simulink model "mrefrobotarm_modified_previous_y_previous_u_previous_ref_prepro"  (R2018b)
settings: Solver=FixedStepAuto  StartTime=0.0  StopTime=10  RelTol=1e-3  AbsTol=1e-6
undefined symbols (not defined in the file or in its folder): cc, options
libraries: neural x594, simulink x1
(part 10 of 22)

== system mrefrobotarm_modified_previous_y_previous_u_previous_ref_prepro/pre_0.00001/Layer 3/Delays 1 ==
  "p{3}" : Inport  PortDimensions=30
      mask Display: e = 0.06;c1 = [120 230 180]/255;c2 = ([120 230 180]+0)/(256+128);c3 = ([120 230 180]+128)/(256+128);patch([0 1 1 0],[0 0 1 1],c1);patch([0 1 1 1-e 1-e 0+e],[0 0 1 1-e 0+e 0+e],c2);patch([0 0 1 1-e 0+e 0+e],[0 1 1 1-e 1-e 0+e],c3);plot([0 1 1 0 0],[0 0 1 1 0]);
  mux : Mux  Inputs=1
      mask Display: e = 0.06;c1 = [120 150 230]/255;c2 = ([120 150 230]+0)/383;c3 = ([120 150 230]+128)/383;patch([0 1 1 0],[0 0 1 1],c1);patch([0 1 1 1-e 1-e 0+e],[0 0 1 1-e 0+e 0+e],c2);patch([0 0 1 1-e 0+e 0+e],[0 1 1 1-e 1-e 0+e],c3);plot([0 1 1 0 0],[0 0 1 1 0]);disp('Mux')
  "pd{3,2}" : Outport
      mask Display: e = 0.06;c1 = [120 230 180]/255;c2 = ([120 230 180]+0)/(256+128);c3 = ([120 230 180]+128)/(256+128);patch([0 1 1 0],[0 0 1 1],c1);patch([0 1 1 1-e 1-e 0+e],[0 0 1 1-e 0+e 0+e],c2);patch([0 0 1 1-e 0+e 0+e],[0 1 1 1-e 1-e 0+e],c3);plot([0 1 1 0 0],[0 0 1 1 0]);
  wires:
  "p{3}"/1 -> mux/1
  mux/1 -> "pd{3,2}"/1

== system mrefrobotarm_modified_previous_y_previous_u_previous_ref_prepro/pre_0.00001/Layer 3/LW{3,2} ==
  "ad{3,2}" : Inport  PortDimensions=30
      mask Display: e = 0.06;c1 = [120 230 180]/255;c2 = ([120 230 180]+0)/(256+128);c3 = ([120 230 180]+128)/(256+128);patch([0 1 1 0],[0 0 1 1],c1);patch([0 1 1 1-e 1-e 0+e],[0 0 1 1-e 0+e 0+e],c2);patch([0 0 1 1-e 0+e 0+e],[0 1 1 1-e 1-e 0+e],c3);plot([0 1 1 0 0],[0 0 1 1 0]);
  "IW{3,2}(1,:)'" : Constant  Value=[-0.02708099117104183217730195565309259109199047088623046875;-0.036414425339180954421802738352198502980172634124755859375;-0.53579786648775529211974344434565864503383636474609375;0.11467219823347153673243070670650922693312168121337890625;0.460121219342909448801748339974437840282917022705078125;-0.355936329943013329835110880594584159553050994873046875;-0.14997445769222839118128831614740192890167236328125;-0.401359794727670859959545168749173171818256378173828125;0.012080379935268614755017324569053016602993011474609375;-0.0298262408680656510018280869189766235649585723876953125;-0.30471843862437941741205804646597243845462799072265625;0.1635094519253192657526341236007283441722393035888671875;-0.322365045322164756047556011253618635237216949462890625;0.2441242607764374794587780570509494282305240631103515625;0.05360123386870309369900411411435925401747226715087890625;0.048342927129308037315080781581855262629687786102294921875;0.4674318676620703438828741127508692443370819091796875;-0.11851143462209069723289900366580695845186710357666015625;0.14037975115201273279552651729318313300609588623046875;-0.415865215452181635757966660094098187983036041259765625;-0.42716646209657971322570801930851303040981292724609375;-0.381889610047790262203903921545133925974369049072265625;0.145833587060073599506182517870911397039890289306640625;-0.2441832694725563357440734080228139646351337432861328125;-0.22157671356331276601991930874646641314029693603515625;0.319918117660031697813138862329651601612567901611328125;-0.528575828850534445990660969982855021953582763671875;-0.417695234753292510276878601871430873870849609375;-0.0213015001949658951130306405730152619071304798126220703125;-0.427062730500115728116128366309567354619503021240234375]
      mask Display: e = 0.06;c1 = [120 150 230]/255;c2 = ([120 150 230]+0)/383;c3 = ([120 150 230]+128)/383;patch([0 1 1 0],[0 0 1 1],c1);patch([0 1 1 1-e 1-e 0+e],[0 0 1 1-e 0+e 0+e],c2);patch([0 0 1 1-e 0+e 0+e],[0 1 1 1-e 1-e 0+e],c3);plot([0 1 1 0 0],[0 0 1 1 0]);disp('weights');
  Mux : Mux  Inputs=1
      mask Display: e = 0.06;c1 = [120 150 230]/255;c2 = ([120 150 230]+0)/383;c3 = ([120 150 230]+128)/383;patch([0 1 1 0],[0 0 1 1],c1);patch([0 1 1 1-e 1-e 0+e],[0 0 1 1-e 0+e 0+e],c2);patch([0 0 1 1-e 0+e 0+e],[0 1 1 1-e 1-e 0+e],c3);plot([0 1 1 0 0],[0 0 1 1 0]);disp('Mux');
  dotprod1 : neural/Weight Functions/dotprod
  "lz{3,2}" : Outport
      mask Display: e = 0.06;c1 = [120 230 180]/255;c2 = ([120 230 180]+0)/(256+128);c3 = ([120 230 180]+128)/(256+128);patch([0 1 1 0],[0 0 1 1],c1);patch([0 1 1 1-e 1-e 0+e],[0 0 1 1-e 0+e 0+e],c2);patch([0 0 1 1-e 0+e 0+e],[0 1 1 1-e 1-e 0+e],c3);plot([0 1 1 0 0],[0 0 1 1 0]);
  wires:
  "IW{3,2}(1,:)'"/1 -> dotprod1/1
  "ad{3,2}"/1 -> dotprod1/2
  dotprod1/1 -> Mux/1
  Mux/1 -> "lz{3,2}"/1

== system mrefrobotarm_modified_previous_y_previous_u_previous_ref_prepro/pre_0.00002/Layer 1/Delays 1 ==
  "p{1}" : Inport  PortDimensions=10
      mask Display: e = 0.06;c1 = [120 230 180]/255;c2 = ([120 230 180]+0)/(256+128);c3 = ([120 230 180]+128)/(256+128);patch([0 1 1 0],[0 0 1 1],c1);patch([0 1 1 1-e 1-e 0+e],[0 0 1 1-e 0+e 0+e],c2);patch([0 0 1 1-e 0+e 0+e],[0 1 1 1-e 1-e 0+e],c3);plot([0 1 1 0 0],[0 0 1 1 0]);
  mux : Mux  Inputs=1
      mask Display: e = 0.06;c1 = [120 150 230]/255;c2 = ([120 150 230]+0)/383;c3 = ([120 150 230]+128)/383;patch([0 1 1 0],[0 0 1 1],c1);patch([0 1 1 1-e 1-e 0+e],[0 0 1 1-e 0+e 0+e],c2);patch([0 0 1 1-e 0+e 0+e],[0 1 1 1-e 1-e 0+e],c3);plot([0 1 1 0 0],[0 0 1 1 0]);disp('Mux')
  "pd{1,1}" : Outport
      mask Display: e = 0.06;c1 = [120 230 180]/255;c2 = ([120 230 180]+0)/(256+128);c3 = ([120 230 180]+128)/(256+128);patch([0 1 1 0],[0 0 1 1],c1);patch([0 1 1 1-e 1-e 0+e],[0 0 1 1-e 0+e 0+e],c2);patch([0 0 1 1-e 0+e 0+e],[0 1 1 1-e 1-e 0+e],c3);plot([0 1 1 0 0],[0 0 1 1 0]);
  wires:
  "p{1}"/1 -> mux/1
  mux/1 -> "pd{1,1}"/1

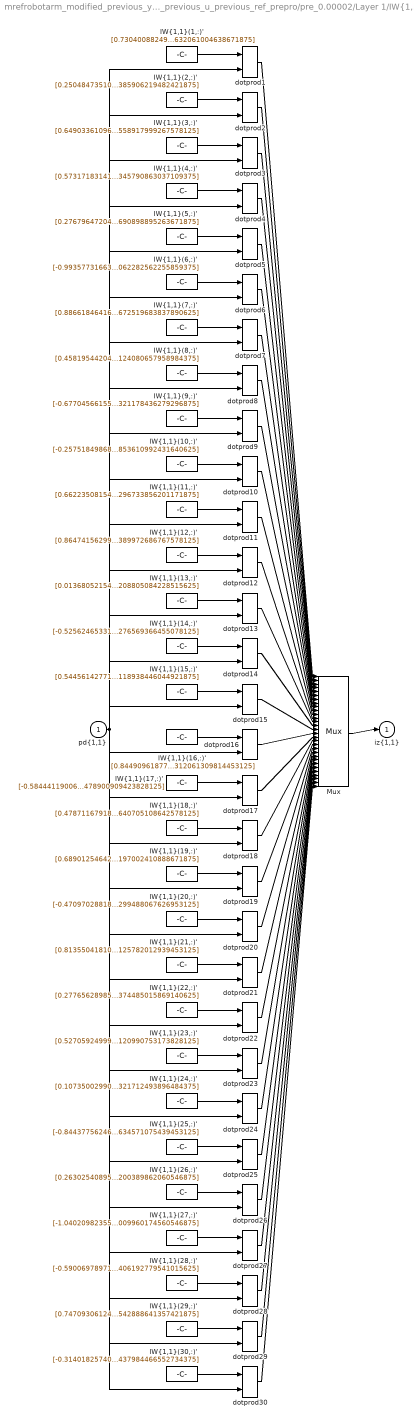
== system mrefrobotarm_modified_previous_y_previous_u_previous_ref_prepro/pre_0.00002/Layer 1/IW{1,1} ==
  "pd{1,1}" : Inport  PortDimensions=10
      mask Display: e = 0.06;c1 = [120 230 180]/255;c2 = ([120 230 180]+0)/(256+128);c3 = ([120 230 180]+128)/(256+128);patch([0 1 1 0],[0 0 1 1],c1);patch([0 1 1 1-e 1-e 0+e],[0 0 1 1-e 0+e 0+e],c2);patch([0 0 1 1-e 0+e 0+e],[0 1 1 1-e 1-e 0+e],c3);plot([0 1 1 0 0],[0 0 1 1 0]);
  "IW{1,1}(1,:)'" : Constant  Value=[0.7304008824925178888776144958683289587497711181640625;0.55735729031188718796130388000165112316608428955078125;-0.274224224023352614043602670790278352797031402587890625;-0.622697954402676057128473985358141362667083740234375;1.191884331831804200163560381042771041393280029296875;-0.67258994734308907847974978722049854695796966552734375;-0.6783417737224137766816056682728230953216552734375;-0.246919049844299520746204734678030945360660552978515625;-0.61337591608532349152227425292949192225933074951171875;-0.60088279688646906162574623522232286632061004638671875]
      mask Display: e = 0.06;c1 = [120 150 230]/255;c2 = ([120 150 230]+0)/383;c3 = ([120 150 230]+128)/383;patch([0 1 1 0],[0 0 1 1],c1);patch([0 1 1 1-e 1-e 0+e],[0 0 1 1-e 0+e 0+e],c2);patch([0 0 1 1-e 0+e 0+e],[0 1 1 1-e 1-e 0+e],c3);plot([0 1 1 0 0],[0 0 1 1 0]);disp('Weights');
  "IW{1,1}(10,:)'" : Constant  Value=[-0.257518498683862950837664129721815697848796844482421875;-0.11405027507294308863894372052527614869177341461181640625;-0.4519201843110665084424226733972318470478057861328125;-0.384415211671115641944851404332439415156841278076171875;-0.356503517164612981904525668142014183104038238525390625;0.9258507361392871448657615474076010286808013916015625;-0.86655442230715185036871162083116360008716583251953125;0.61431897984137495694056951833772473037242889404296875;0.458598179542420825161030961680808104574680328369140625;0.4425235678833419061817266992875374853610992431640625]
      mask Display: e = 0.06;c1 = [120 150 230]/255;c2 = ([120 150 230]+0)/383;c3 = ([120 150 230]+128)/383;patch([0 1 1 0],[0 0 1 1],c1);patch([0 1 1 1-e 1-e 0+e],[0 0 1 1-e 0+e 0+e],c2);patch([0 0 1 1-e 0+e 0+e],[0 1 1 1-e 1-e 0+e],c3);plot([0 1 1 0 0],[0 0 1 1 0]);disp('Weights');
  "IW{1,1}(11,:)'" : Constant  Value=[0.66223508154602706010649626477970741689205169677734375;-0.448412675292931994786016502985148690640926361083984375;0.83225908909172952032662351484759710729122161865234375;0.426264912161532449896839125358383171260356903076171875;0.6714719379842970514715716490172781050205230712890625;-0.5465042912343280878673112965770997107028961181640625;-0.05809258706369181679551871866351575590670108795166015625;-0.8415470336572987708478876811568625271320343017578125;-0.65915992475788309779005658128880895674228668212890625;-0.11957509036706519267578840981514076702296733856201171875]
      mask Display: e = 0.06;c1 = [120 150 230]/255;c2 = ([120 150 230]+0)/383;c3 = ([120 150 230]+128)/383;patch([0 1 1 0],[0 0 1 1],c1);patch([0 1 1 1-e 1-e 0+e],[0 0 1 1-e 0+e 0+e],c2);patch([0 0 1 1-e 0+e 0+e],[0 1 1 1-e 1-e 0+e],c3);plot([0 1 1 0 0],[0 0 1 1 0]);disp('Weights');
  "IW{1,1}(12,:)'" : Constant  Value=[0.8647415629915180534936780532007105648517608642578125;0.367581229875802384388094878886477090418338775634765625;-0.59028723730554644166801381288678385317325592041015625;-0.62213624516392174168544215717702172696590423583984375;-0.623824016499044287087372140376828610897064208984375;0.504078517565071049233438316150568425655364990234375;-0.70493815736031162355601509261759929358959197998046875;-0.66348746327245378129333630567998625338077545166015625;0.28462536860450959874668797056074254214763641357421875;-0.03806284371844066705126152783122961409389972686767578125]
      mask Display: e = 0.06;c1 = [120 150 230]/255;c2 = ([120 150 230]+0)/383;c3 = ([120 150 230]+128)/383;patch([0 1 1 0],[0 0 1 1],c1);patch([0 1 1 1-e 1-e 0+e],[0 0 1 1-e 0+e 0+e],c2);patch([0 0 1 1-e 0+e 0+e],[0 1 1 1-e 1-e 0+e],c3);plot([0 1 1 0 0],[0 0 1 1 0]);disp('Weights');
  "IW{1,1}(13,:)'" : Constant  Value=[0.0136805215469812425921336540568518103100359439849853515625;-0.34441505779833148093160843927762471139430999755859375;1.0216982880331426652986692715785466134548187255859375;0.2435027042613311099028550188450026325881481170654296875;0.34766871164740809074800154121476225554943084716796875;0.624162933978758882602733137900941073894500732421875;0.6576120651417929341420176569954492151737213134765625;0.7039052895761155337339687321218661963939666748046875;-0.6525688408982965871274473101948387920856475830078125;-0.77884807903645114635082791210152208805084228515625]
      mask Display: e = 0.06;c1 = [120 150 230]/255;c2 = ([120 150 230]+0)/383;c3 = ([120 150 230]+128)/383;patch([0 1 1 0],[0 0 1 1],c1);patch([0 1 1 1-e 1-e 0+e],[0 0 1 1-e 0+e 0+e],c2);patch([0 0 1 1-e 0+e 0+e],[0 1 1 1-e 1-e 0+e],c3);plot([0 1 1 0 0],[0 0 1 1 0]);disp('Weights');
  "IW{1,1}(14,:)'" : Constant  Value=[-0.5256246533137678422775707076652906835079193115234375;0.7114248951113688601566309444024227559566497802734375;0.75946178060658031672147671997663564980030059814453125;0.488034362594031267956751207748311571776866912841796875;0.307774644334204150464273652687552385032176971435546875;1.17777346771161273153438742156140506267547607421875;-1.060571928032192801083510858006775379180908203125;-0.8649891627355097423190954941674135625362396240234375;-0.07488935386397999049989948616712354123592376708984375;0.47549822229369731463322068520938046276569366455078125]
      mask Display: e = 0.06;c1 = [120 150 230]/255;c2 = ([120 150 230]+0)/383;c3 = ([120 150 230]+128)/383;patch([0 1 1 0],[0 0 1 1],c1);patch([0 1 1 1-e 1-e 0+e],[0 0 1 1-e 0+e 0+e],c2);patch([0 0 1 1-e 0+e 0+e],[0 1 1 1-e 1-e 0+e],c3);plot([0 1 1 0 0],[0 0 1 1 0]);disp('Weights');
  "IW{1,1}(15,:)'" : Constant  Value=[0.54456142771591242723872028363985009491443634033203125;0.1924337675434008299024668531274073757231235504150390625;0.1103372802512005979025389024172909557819366455078125;0.366407819941435786148531406070105731487274169921875;2.13415426335682933967063945601694285869598388671875;-1.571152442476574151442036963999271392822265625;0.87951877890999152764806012783083133399486541748046875;0.059551333168809457430104004060922306962311267852783203125;0.06808296663973219253751523183382232673466205596923828125;0.31540879799017040863162719688261859118938446044921875]
      mask Display: e = 0.06;c1 = [120 150 230]/255;c2 = ([120 150 230]+0)/383;c3 = ([120 150 230]+128)/383;patch([0 1 1 0],[0 0 1 1],c1);patch([0 1 1 1-e 1-e 0+e],[0 0 1 1-e 0+e 0+e],c2);patch([0 0 1 1-e 0+e 0+e],[0 1 1 1-e 1-e 0+e],c3);plot([0 1 1 0 0],[0 0 1 1 0]);disp('Weights');
  "IW{1,1}(16,:)'" : Constant  Value=[0.8449096187701414795157006665249355137348175048828125;-0.74746261915909906203836499116732738912105560302734375;0.329952307077657158718153596055344678461551666259765625;0.8260485994065922543683200274244882166385650634765625;0.54075535587794931746685733742197044193744659423828125;1.7436566173639054255772862234152853488922119140625;-0.1463094264313840875413319508879794739186763763427734375;-0.660820573047626425022826879285275936126708984375;-0.06815574103313228049305649847156018950045108795166015625;0.42592880572693747609491765615530312061309814453125]
      mask Display: e = 0.06;c1 = [120 150 230]/255;c2 = ([120 150 230]+0)/383;c3 = ([120 150 230]+128)/383;patch([0 1 1 0],[0 0 1 1],c1);patch([0 1 1 1-e 1-e 0+e],[0 0 1 1-e 0+e 0+e],c2);patch([0 0 1 1-e 0+e 0+e],[0 1 1 1-e 1-e 0+e],c3);plot([0 1 1 0 0],[0 0 1 1 0]);disp('Weights');
  "IW{1,1}(17,:)'" : Constant  Value=[-0.58444119006608763466914524542517028748989105224609375;-0.80689482797726075347100049839355051517486572265625;-0.21128881566034196648473653112887404859066009521484375;0.1993104800768525641796458103272016160190105438232421875;0.7910371685352901582888307530083693563938140869140625;-1.6374659717699844296845412827678956091403961181640625;0.2347058211055967069658123591580078937113285064697265625;-0.316128742752765978796247736681834794580936431884765625;0.0220931580819457261399829661741023301146924495697021484375;0.50710898397081038968536859101732261478900909423828125]
      mask Display: e = 0.06;c1 = [120 150 230]/255;c2 = ([120 150 230]+0)/383;c3 = ([120 150 230]+128)/383;patch([0 1 1 0],[0 0 1 1],c1);patch([0 1 1 1-e 1-e 0+e],[0 0 1 1-e 0+e 0+e],c2);patch([0 0 1 1-e 0+e 0+e],[0 1 1 1-e 1-e 0+e],c3);plot([0 1 1 0 0],[0 0 1 1 0]);disp('Weights');
  "IW{1,1}(18,:)'" : Constant  Value=[0.478711679183998206621453164189006201922893524169921875;-0.6843316515233277552709978408529423177242279052734375;0.58763716442424451802395424238056875765323638916015625;0.67534649893978448975673245513462461531162261962890625;-1.089531552775316658454585194704122841358184814453125;1.1625260678634479205584284500218927860260009765625;0.58469035382791589849915681043057702481746673583984375;0.10013888820124013101509063972116564400494098663330078125;-0.78463798649333116319581904463120736181735992431640625;-0.65112497301214411482561672528390772640705108642578125]
      mask Display: e = 0.06;c1 = [120 150 230]/255;c2 = ([120 150 230]+0)/383;c3 = ([120 150 230]+128)/383;patch([0 1 1 0],[0 0 1 1],c1);patch([0 1 1 1-e 1-e 0+e],[0 0 1 1-e 0+e 0+e],c2);patch([0 0 1 1-e 0+e 0+e],[0 1 1 1-e 1-e 0+e],c3);plot([0 1 1 0 0],[0 0 1 1 0]);disp('Weights');
  "IW{1,1}(19,:)'" : Constant  Value=[0.689012546428803052123157613095827400684356689453125;-0.047229633595688429170689204283917206339538097381591796875;-0.7243675903009723082703885665978305041790008544921875;0.1993048568244606411070662943529896438121795654296875;-0.31650746445339195123125364261795766651630401611328125;0.822948088279580769466292622382752597332000732421875;0.98922181344819126724843272313592024147510528564453125;0.440776909161637975298475566887645982205867767333984375;-0.88029002172244386059674070565961301326751708984375;-0.314501274632482619164619563889573328197002410888671875]
      mask Display: e = 0.06;c1 = [120 150 230]/255;c2 = ([120 150 230]+0)/383;c3 = ([120 150 230]+128)/383;patch([0 1 1 0],[0 0 1 1],c1);patch([0 1 1 1-e 1-e 0+e],[0 0 1 1-e 0+e 0+e],c2);patch([0 0 1 1-e 0+e 0+e],[0 1 1 1-e 1-e 0+e],c3);plot([0 1 1 0 0],[0 0 1 1 0]);disp('Weights');
  "IW{1,1}(2,:)'" : Constant  Value=[0.25048473510027247090903301796060986816883087158203125;-1.0819345400682920388391039523412473499774932861328125;0.84795876175950513076173820081748999655246734619140625;-0.56312297055498350406566032688715495169162750244140625;-0.45823196200243498932280772351077757775783538818359375;0.1609611189829285304853101479238830506801605224609375;0.9208277384343850346937188078300096094608306884765625;0.046244571997199612756190845175296999514102935791015625;0.7151359877845873125323805652442388236522674560546875;-0.363929879968436231774120415138895623385906219482421875]
      mask Display: e = 0.06;c1 = [120 150 230]/255;c2 = ([120 150 230]+0)/383;c3 = ([120 150 230]+128)/383;patch([0 1 1 0],[0 0 1 1],c1);patch([0 1 1 1-e 1-e 0+e],[0 0 1 1-e 0+e 0+e],c2);patch([0 0 1 1-e 0+e 0+e],[0 1 1 1-e 1-e 0+e],c3);plot([0 1 1 0 0],[0 0 1 1 0]);disp('Weights');
  "IW{1,1}(20,:)'" : Constant  Value=[-0.47097028818942165973027158543118275701999664306640625;0.74309036858321697582852038976852782070636749267578125;-0.553976745551350457930084303370676934719085693359375;0.033889115275527535720012650699572986923158168792724609375;0.364869656293961508453094211290590465068817138671875;0.410145163811602930792332699638791382312774658203125;-0.2345107364438836217157557939572143368422985076904296875;-0.54322703205234412759949691462679766118526458740234375;0.1590784487766848942502662112019606865942478179931640625;-0.383833262476066583435141410518554039299488067626953125]
      mask Display: e = 0.06;c1 = [120 150 230]/255;c2 = ([120 150 230]+0)/383;c3 = ([120 150 230]+128)/383;patch([0 1 1 0],[0 0 1 1],c1);patch([0 1 1 1-e 1-e 0+e],[0 0 1 1-e 0+e 0+e],c2);patch([0 0 1 1-e 0+e 0+e],[0 1 1 1-e 1-e 0+e],c3);plot([0 1 1 0 0],[0 0 1 1 0]);disp('Weights');
  "IW{1,1}(21,:)'" : Constant  Value=[0.81355041810238504229602085615624673664569854736328125;-1.1474633075534554915719809287111274898052215576171875;0.796433568812742631592982434085570275783538818359375;-0.53342796022723260040976356322062201797962188720703125;0.2163303690425346648140703109675087034702301025390625;-0.053740994151761929675803486361473915167152881622314453125;-0.7139248086813463345379204838536679744720458984375;-0.36399888500070876062864044797606766223907470703125;0.6045317614051251009499310384853743016719818115234375;0.08818159555106726277262652047284063883125782012939453125]
      mask Display: e = 0.06;c1 = [120 150 230]/255;c2 = ([120 150 230]+0)/383;c3 = ([120 150 230]+128)/383;patch([0 1 1 0],[0 0 1 1],c1);patch([0 1 1 1-e 1-e 0+e],[0 0 1 1-e 0+e 0+e],c2);patch([0 0 1 1-e 0+e 0+e],[0 1 1 1-e 1-e 0+e],c3);plot([0 1 1 0 0],[0 0 1 1 0]);disp('Weights');
  "IW{1,1}(22,:)'" : Constant  Value=[0.2776562898561787395834699054830707609653472900390625;-1.2287554150803090546872908817022107541561126708984375;0.0209047426415454491721579444174494710750877857208251953125;0.000445490992757326966476616458834314471459947526454925537109375;1.0480957638323007419245413984754122793674468994140625;-0.07403841976945002567589426689664833247661590576171875;-0.37438154479052376810699342968291603028774261474609375;-0.52846064882596965883720940837520174682140350341796875;0.415750687036309296562563986299210228025913238525390625;0.85104284168978028279894942897954024374485015869140625]
      mask Display: e = 0.06;c1 = [120 150 230]/255;c2 = ([120 150 230]+0)/383;c3 = ([120 150 230]+128)/383;patch([0 1 1 0],[0 0 1 1],c1);patch([0 1 1 1-e 1-e 0+e],[0 0 1 1-e 0+e 0+e],c2);patch([0 0 1 1-e 0+e 0+e],[0 1 1 1-e 1-e 0+e],c3);plot([0 1 1 0 0],[0 0 1 1 0]);disp('Weights');
  "IW{1,1}(23,:)'" : Constant  Value=[0.52705924999088493709820113508612848818302154541015625;0.0660054220044097583741660173473064787685871124267578125;-1.36875726794443952627489125006832182407379150390625;0.311968753379823604543474857564433477818965911865234375;-0.46009367922534283312785419184365309774875640869140625;-0.481466025254796925469946700104628689587116241455078125;-0.3329466073938880388283223510370589792728424072265625;0.1974229762788315689636675642759655602276325225830078125;-1.1254391851952505465561671371688134968280792236328125;-0.9640440286026532579199965766747482120990753173828125]
      mask Display: e = 0.06;c1 = [120 150 230]/255;c2 = ([120 150 230]+0)/383;c3 = ([120 150 230]+128)/383;patch([0 1 1 0],[0 0 1 1],c1);patch([0 1 1 1-e 1-e 0+e],[0 0 1 1-e 0+e 0+e],c2);patch([0 0 1 1-e 0+e 0+e],[0 1 1 1-e 1-e 0+e],c3);plot([0 1 1 0 0],[0 0 1 1 0]);disp('Weights');
  "IW{1,1}(24,:)'" : Constant  Value=[0.10735002990849211446100497369116055779159069061279296875;0.1288206058417812605032537476290599443018436431884765625;0.788111618675113145826571781071834266185760498046875;0.64028048347422850117283132931333966553211212158203125;-0.433917129931848444268638331777765415608882904052734375;0.5940663745965399922255301135010085999965667724609375;1.12816027899131920975150933372788131237030029296875;0.112385069453518282589499222012818790972232818603515625;0.024179242542832761475590785948952543549239635467529296875;0.463315765300100268486716004190384410321712493896484375]
      mask Display: e = 0.06;c1 = [120 150 230]/255;c2 = ([120 150 230]+0)/383;c3 = ([120 150 230]+128)/383;patch([0 1 1 0],[0 0 1 1],c1);patch([0 1 1 1-e 1-e 0+e],[0 0 1 1-e 0+e 0+e],c2);patch([0 0 1 1-e 0+e 0+e],[0 1 1 1-e 1-e 0+e],c3);plot([0 1 1 0 0],[0 0 1 1 0]);disp('Weights');
  "IW{1,1}(25,:)'" : Constant  Value=[-0.84437756246050066355479657431715168058872222900390625;-0.0846648540292919415950478878585272468626499176025390625;0.18704027349657670331595227253274060785770416259765625;-0.2898728359229156836818219744600355625152587890625;-1.09397119609031445719438124797306954860687255859375;-0.44686289863698658297863630650681443512439727783203125;-0.89946061161813783968455027206800878047943115234375;0.636115631845411311218185801408253610134124755859375;0.061844671970694618801100972405038191936910152435302734375;0.17568172897040501556631397761520929634571075439453125]
      mask Display: e = 0.06;c1 = [120 150 230]/255;c2 = ([120 150 230]+0)/383;c3 = ([120 150 230]+128)/383;patch([0 1 1 0],[0 0 1 1],c1);patch([0 1 1 1-e 1-e 0+e],[0 0 1 1-e 0+e 0+e],c2);patch([0 0 1 1-e 0+e 0+e],[0 1 1 1-e 1-e 0+e],c3);plot([0 1 1 0 0],[0 0 1 1 0]);disp('Weights');
  "IW{1,1}(26,:)'" : Constant  Value=[0.26302540895656945085789857330382801592350006103515625;-0.3606987416329634488221245192107744514942169189453125;-0.52244731928137699838998742052353918552398681640625;-0.0285817138234593405565764356879299157299101352691650390625;-0.436131655659286410209318773922859691083431243896484375;1.1469446426500125024716680854908190667629241943359375;0.80450112209670876506351078205625526607036590576171875;0.30490732299961365026064186167786829173564910888671875;-0.50300669421127974789698100721579976379871368408203125;-0.71714061620181535072759970717015676200389862060546875]
      mask Display: e = 0.06;c1 = [120 150 230]/255;c2 = ([120 150 230]+0)/383;c3 = ([120 150 230]+128)/383;patch([0 1 1 0],[0 0 1 1],c1);patch([0 1 1 1-e 1-e 0+e],[0 0 1 1-e 0+e 0+e],c2);patch([0 0 1 1-e 0+e 0+e],[0 1 1 1-e 1-e 0+e],c3);plot([0 1 1 0 0],[0 0 1 1 0]);disp('Weights');
  "IW{1,1}(27,:)'" : Constant  Value=[-1.040209823554227863695587075199000537395477294921875;0.2194302039461969167088994936420931480824947357177734375;-0.528908307700870050638286556932143867015838623046875;-0.478955296274611808104992860535276122391223907470703125;1.0535535961804505244998608759487979114055633544921875;0.1624369124767082173121934829396195709705352783203125;-0.4332507443024322668634340516291558742523193359375;-0.104280016056704283311518111077020876109600067138671875;-0.73485800356468755634153922073892317712306976318359375;-0.50523587261920777091717127404990606009960174560546875]
      mask Display: e = 0.06;c1 = [120 150 230]/255;c2 = ([120 150 230]+0)/383;c3 = ([120 150 230]+128)/383;patch([0 1 1 0],[0 0 1 1],c1);patch([0 1 1 1-e 1-e 0+e],[0 0 1 1-e 0+e 0+e],c2);patch([0 0 1 1-e 0+e 0+e],[0 1 1 1-e 1-e 0+e],c3);plot([0 1 1 0 0],[0 0 1 1 0]);disp('Weights');
  "IW{1,1}(28,:)'" : Constant  Value=[-0.5900697897165836369737235145294107496738433837890625;0.76162907946809366155349607652169652283191680908203125;0.41444551213807889755713631529943086206912994384765625;0.2475855026572744421731187003388185985386371612548828125;0.66626814957252367133122561426716856658458709716796875;-0.60986312197679648505754812504164874553680419921875;-0.66349745726455811034583120999741367995738983154296875;1.0245903704451977400680107166408561170101165771484375;0.07942192957857995005976903257760568521916866302490234375;0.60212820522696175462584733395488001406192779541015625]
      mask Display: e = 0.06;c1 = [120 150 230]/255;c2 = ([120 150 230]+0)/383;c3 = ([120 150 230]+128)/383;patch([0 1 1 0],[0 0 1 1],c1);patch([0 1 1 1-e 1-e 0+e],[0 0 1 1-e 0+e 0+e],c2);patch([0 0 1 1-e 0+e 0+e],[0 1 1 1-e 1-e 0+e],c3);plot([0 1 1 0 0],[0 0 1 1 0]);disp('Weights');
  "IW{1,1}(29,:)'" : Constant  Value=[0.74709306124852636887823109645978547632694244384765625;-0.1787623438079971316394534142091288231313228607177734375;0.71059062589504484730440481143887154757976531982421875;-0.0764085424701572424321938115099328570067882537841796875;-0.68254969580245850035993271376355551183223724365234375;-0.27645474241165579609713631725753657519817352294921875;0.7957867559310898286639712750911712646484375;-0.310195487014007176274077437483356334269046783447265625;-0.08741571691373951902281902448521577753126621246337890625;0.64349518684717121885796586866490542888641357421875]
      mask Display: e = 0.06;c1 = [120 150 230]/255;c2 = ([120 150 230]+0)/383;c3 = ([120 150 230]+128)/383;patch([0 1 1 0],[0 0 1 1],c1);patch([0 1 1 1-e 1-e 0+e],[0 0 1 1-e 0+e 0+e],c2);patch([0 0 1 1-e 0+e 0+e],[0 1 1 1-e 1-e 0+e],c3);plot([0 1 1 0 0],[0 0 1 1 0]);disp('Weights');
  "IW{1,1}(3,:)'" : Constant  Value=[0.64903361096156964027414915108238346874713897705078125;0.437019374876214505842852986461366526782512664794921875;-0.167251601072769318090394108367036096751689910888671875;-0.31406238658746177261349430409609340131282806396484375;0.58805134800320446597510226638405583798885345458984375;-0.278110750553261787398895421574707143008708953857421875;0.6085357582623387440179385521332733333110809326171875;-0.88598878541688963483835550505318678915500640869140625;0.55934294191945366225837688034516759216785430908203125;-0.7817235337581742715684640643303282558917999267578125]
      mask Display: e = 0.06;c1 = [120 150 230]/255;c2 = ([120 150 230]+0)/383;c3 = ([120 150 230]+128)/383;patch([0 1 1 0],[0 0 1 1],c1);patch([0 1 1 1-e 1-e 0+e],[0 0 1 1-e 0+e 0+e],c2);patch([0 0 1 1-e 0+e 0+e],[0 1 1 1-e 1-e 0+e],c3);plot([0 1 1 0 0],[0 0 1 1 0]);disp('Weights');
  "IW{1,1}(30,:)'" : Constant  Value=[-0.314018257403796408055995925678871572017669677734375;1.0177950132940696281735881711938418447971343994140625;0.0337987857613381847965428050883929245173931121826171875;-0.5754491029841373173070451230159960687160491943359375;0.9657995086592559008664693465107120573520660400390625;-0.0098118034820728998457450842352045583538711071014404296875;-0.55853197033475232569088575473870150744915008544921875;0.54986807670145954052287606828031130135059356689453125;-0.235245471913925030538194960172404535114765167236328125;0.49020379140686054508790903128101490437984466552734375]
      mask Display: e = 0.06;c1 = [120 150 230]/255;c2 = ([120 150 230]+0)/383;c3 = ([120 150 230]+128)/383;patch([0 1 1 0],[0 0 1 1],c1);patch([0 1 1 1-e 1-e 0+e],[0 0 1 1-e 0+e 0+e],c2);patch([0 0 1 1-e 0+e 0+e],[0 1 1 1-e 1-e 0+e],c3);plot([0 1 1 0 0],[0 0 1 1 0]);disp('Weights');
  "IW{1,1}(4,:)'" : Constant  Value=[0.57317183141110883415336729740374721586704254150390625;-0.1558520380054415344073248661516117863357067108154296875;0.71893072814568304007565302526927553117275238037109375;0.5056102505369846067395656064036302268505096435546875;1.472839369471885984097525579272769391536712646484375;0.86104308527801187711503416721825487911701202392578125;0.2270019911193220940592851775363669730722904205322265625;0.357781543772290933080881814021267928183078765869140625;-0.7114765167660632716462032476556487381458282470703125;-0.361173298051945257380879183983779512345790863037109375]
      mask Display: e = 0.06;c1 = [120 150 230]/255;c2 = ([120 150 230]+0)/383;c3 = ([120 150 230]+128)/383;patch([0 1 1 0],[0 0 1 1],c1);patch([0 1 1 1-e 1-e 0+e],[0 0 1 1-e 0+e 0+e],c2);patch([0 0 1 1-e 0+e 0+e],[0 1 1 1-e 1-e 0+e],c3);plot([0 1 1 0 0],[0 0 1 1 0]);disp('Weights');
  "IW{1,1}(5,:)'" : Constant  Value=[0.27679647204057411524757981169386766850948333740234375;-0.448323161483788645842452069700811989605426788330078125;-0.84154234253909532270654381136409938335418701171875;0.2093410037801492762365995758955250494182109832763671875;1.33079770660296592410531957284547388553619384765625;-0.64926906407087814354639476732700131833553314208984375;-0.437686617135825184465858228577417321503162384033203125;0.6736944795738519786709730396978557109832763671875;0.486424352859251618586000631694332696497440338134765625;0.52492210464086042076559124325285665690898895263671875]
      mask Display: e = 0.06;c1 = [120 150 230]/255;c2 = ([120 150 230]+0)/383;c3 = ([120 150 230]+128)/383;patch([0 1 1 0],[0 0 1 1],c1);patch([0 1 1 1-e 1-e 0+e],[0 0 1 1-e 0+e 0+e],c2);patch([0 0 1 1-e 0+e 0+e],[0 1 1 1-e 1-e 0+e],c3);plot([0 1 1 0 0],[0 0 1 1 0]);disp('Weights');
  "IW{1,1}(6,:)'" : Constant  Value=[-0.993577316638220242595025410992093384265899658203125;0.26861453719231465075978348977514542639255523681640625;0.446118986558865504576942839776165783405303955078125;0.00403557737388328917338409240755936480127274990081787109375;0.57898291647205812893162146792747080326080322265625;-0.80893103142543532069197453893139027059078216552734375;0.64470728835652357791019539945409633219242095947265625;-0.58404770040326869917635121964849531650543212890625;0.00332342982215149719549263096496360958553850650787353515625;-1.009575397773443850013563860557042062282562255859375]
      mask Display: e = 0.06;c1 = [120 150 230]/255;c2 = ([120 150 230]+0)/383;c3 = ([120 150 230]+128)/383;patch([0 1 1 0],[0 0 1 1],c1);patch([0 1 1 1-e 1-e 0+e],[0 0 1 1-e 0+e 0+e],c2);patch([0 0 1 1-e 0+e 0+e],[0 1 1 1-e 1-e 0+e],c3);plot([0 1 1 0 0],[0 0 1 1 0]);disp('Weights');
  "IW{1,1}(7,:)'" : Constant  Value=[0.88661846416621015176673381574801169335842132568359375;0.40058986394658224750031649818993173539638519287109375;0.6645161052261083778347483530524186789989471435546875;0.64015798035069948479502954796771518886089324951171875;0.198609264088941361858786649463581852614879608154296875;-0.334286157804024097739414855823270045220851898193359375;-0.77495885273977893614727463500457815825939178466796875;0.5937368738992947481136752685415558516979217529296875;0.6817369876034284903454363302444107830524444580078125;0.258994385290615358741206364356912672519683837890625]
      mask Display: e = 0.06;c1 = [120 150 230]/255;c2 = ([120 150 230]+0)/383;c3 = ([120 150 230]+128)/383;patch([0 1 1 0],[0 0 1 1],c1);patch([0 1 1 1-e 1-e 0+e],[0 0 1 1-e 0+e 0+e],c2);patch([0 0 1 1-e 0+e 0+e],[0 1 1 1-e 1-e 0+e],c3);plot([0 1 1 0 0],[0 0 1 1 0]);disp('Weights');
  "IW{1,1}(8,:)'" : Constant  Value=[0.458195442046004319802676718609291128814220428466796875;0.50866744420029130768767799963825382292270660400390625;-0.143247959120673840072157645408879034221172332763671875;-0.037248813613814345246932902000480680726468563079833984375;-1.21739460049685277454045717604458332061767578125;0.25765485438492763403672825006651692092418670654296875;0.307378207408996073635165657833567820489406585693359375;0.6608603895715390308396308682858943939208984375;0.130263081737165886675455794829758815467357635498046875;-0.890647106531073262658537714742124080657958984375]
      mask Display: e = 0.06;c1 = [120 150 230]/255;c2 = ([120 150 230]+0)/383;c3 = ([120 150 230]+128)/383;patch([0 1 1 0],[0 0 1 1],c1);patch([0 1 1 1-e 1-e 0+e],[0 0 1 1-e 0+e 0+e],c2);patch([0 0 1 1-e 0+e 0+e],[0 1 1 1-e 1-e 0+e],c3);plot([0 1 1 0 0],[0 0 1 1 0]);disp('Weights');
  "IW{1,1}(9,:)'" : Constant  Value=[-0.67704566155669232419000991285429336130619049072265625;0.86987463044085366892232968893949873745441436767578125;0.53946517224805834445078289718367159366607666015625;0.10588155802941863481425599502472323365509510040283203125;0.2165907337617493377823763012202107347548007965087890625;0.72791800497685310578077633181237615644931793212890625;0.1794164031154424632230615088701597414910793304443359375;0.5996025850570474435841106242150999605655670166015625;0.82267452109620708977644198967027477920055389404296875;0.78739881105265030480921950584161095321178436279296875]
      mask Display: e = 0.06;c1 = [120 150 230]/255;c2 = ([120 150 230]+0)/383;c3 = ([120 150 230]+128)/383;patch([0 1 1 0],[0 0 1 1],c1);patch([0 1 1 1-e 1-e 0+e],[0 0 1 1-e 0+e 0+e],c2);patch([0 0 1 1-e 0+e 0+e],[0 1 1 1-e 1-e 0+e],c3);plot([0 1 1 0 0],[0 0 1 1 0]);disp('Weights');
  Mux : Mux  Inputs=30
      mask Display: e = 0.06;c1 = [120 150 230]/255;c2 = ([120 150 230]+0)/383;c3 = ([120 150 230]+128)/383;patch([0 1 1 0],[0 0 1 1],c1);patch([0 1 1 1-e 1-e 0+e],[0 0 1 1-e 0+e 0+e],c2);patch([0 0 1 1-e 0+e 0+e],[0 1 1 1-e 1-e 0+e],c3);plot([0 1 1 0 0],[0 0 1 1 0]);disp('Mux');
  dotprod{1..30} (30 alike) : neural/Weight Functions/dotprod
  "iz{1,1}" : Outport
      mask Display: e = 0.06;c1 = [120 230 180]/255;c2 = ([120 230 180]+0)/(256+128);c3 = ([120 230 180]+128)/(256+128);patch([0 1 1 0],[0 0 1 1],c1);patch([0 1 1 1-e 1-e 0+e],[0 0 1 1-e 0+e 0+e],c2);patch([0 0 1 1-e 0+e 0+e],[0 1 1 1-e 1-e 0+e],c3);plot([0 1 1 0 0],[0 0 1 1 0]);
  wires:
  "IW{1,1}(1,:)'"/1 -> dotprod1/1
  "pd{1,1}"/1 -> dotprod1/2, dotprod2/2, dotprod3/2, dotprod4/2, dotprod5/2, dotprod6/2, dotprod7/2, dotprod8/2, dotprod9/2, dotprod10/2, dotprod11/2, dotprod12/2, dotprod13/2, dotprod14/2, dotprod15/2, dotprod16/2, dotprod17/2, dotprod18/2, dotprod19/2, dotprod20/2, dotprod21/2, dotprod22/2, dotprod23/2, dotprod24/2, dotprod25/2, dotprod26/2, dotprod27/2, dotprod28/2, dotprod29/2, dotprod30/2
  dotprod1/1 -> Mux/1
  "IW{1,1}(2,:)'"/1 -> dotprod2/1
  dotprod2/1 -> Mux/2
  "IW{1,1}(3,:)'"/1 -> dotprod3/1
  dotprod3/1 -> Mux/3
  "IW{1,1}(4,:)'"/1 -> dotprod4/1
  dotprod4/1 -> Mux/4
  "IW{1,1}(5,:)'"/1 -> dotprod5/1
  dotprod5/1 -> Mux/5
  "IW{1,1}(6,:)'"/1 -> dotprod6/1
  dotprod6/1 -> Mux/6
  "IW{1,1}(7,:)'"/1 -> dotprod7/1
  dotprod7/1 -> Mux/7
  "IW{1,1}(8,:)'"/1 -> dotprod8/1
  dotprod8/1 -> Mux/8
  "IW{1,1}(9,:)'"/1 -> dotprod9/1
  dotprod9/1 -> Mux/9
  "IW{1,1}(10,:)'"/1 -> dotprod10/1
  dotprod10/1 -> Mux/10
  "IW{1,1}(11,:)'"/1 -> dotprod11/1
  dotprod11/1 -> Mux/11
  "IW{1,1}(12,:)'"/1 -> dotprod12/1
  dotprod12/1 -> Mux/12
  "IW{1,1}(13,:)'"/1 -> dotprod13/1
  dotprod13/1 -> Mux/13
  "IW{1,1}(14,:)'"/1 -> dotprod14/1
  dotprod14/1 -> Mux/14
  "IW{1,1}(15,:)'"/1 -> dotprod15/1
  dotprod15/1 -> Mux/15
  "IW{1,1}(16,:)'"/1 -> dotprod16/1
  dotprod16/1 -> Mux/16
  "IW{1,1}(17,:)'"/1 -> dotprod17/1
  dotprod17/1 -> Mux/17
  "IW{1,1}(18,:)'"/1 -> dotprod18/1
  dotprod18/1 -> Mux/18
  "IW{1,1}(19,:)'"/1 -> dotprod19/1
  dotprod19/1 -> Mux/19
  "IW{1,1}(20,:)'"/1 -> dotprod20/1
  dotprod20/1 -> Mux/20
  "IW{1,1}(21,:)'"/1 -> dotprod21/1
  dotprod21/1 -> Mux/21
  "IW{1,1}(22,:)'"/1 -> dotprod22/1
  dotprod22/1 -> Mux/22
  "IW{1,1}(23,:)'"/1 -> dotprod23/1
  dotprod23/1 -> Mux/23
  "IW{1,1}(24,:)'"/1 -> dotprod24/1
  dotprod24/1 -> Mux/24
  "IW{1,1}(25,:)'"/1 -> dotprod25/1
  dotprod25/1 -> Mux/25
  "IW{1,1}(26,:)'"/1 -> dotprod26/1
  dotprod26/1 -> Mux/26
  "IW{1,1}(27,:)'"/1 -> dotprod27/1
  dotprod27/1 -> Mux/27
  "IW{1,1}(28,:)'"/1 -> dotprod28/1
  dotprod28/1 -> Mux/28
  "IW{1,1}(29,:)'"/1 -> dotprod29/1
  dotprod29/1 -> Mux/29
  "IW{1,1}(30,:)'"/1 -> dotprod30/1
  dotprod30/1 -> Mux/30
  Mux/1 -> "iz{1,1}"/1

== system mrefrobotarm_modified_previous_y_previous_u_previous_ref_prepro/pre_0.00002/Layer 2/Delays 1 ==
  "p{2}" : Inport  PortDimensions=30
      mask Display: e = 0.06;c1 = [120 230 180]/255;c2 = ([120 230 180]+0)/(256+128);c3 = ([120 230 180]+128)/(256+128);patch([0 1 1 0],[0 0 1 1],c1);patch([0 1 1 1-e 1-e 0+e],[0 0 1 1-e 0+e 0+e],c2);patch([0 0 1 1-e 0+e 0+e],[0 1 1 1-e 1-e 0+e],c3);plot([0 1 1 0 0],[0 0 1 1 0]);
  mux : Mux  Inputs=1
      mask Display: e = 0.06;c1 = [120 150 230]/255;c2 = ([120 150 230]+0)/383;c3 = ([120 150 230]+128)/383;patch([0 1 1 0],[0 0 1 1],c1);patch([0 1 1 1-e 1-e 0+e],[0 0 1 1-e 0+e 0+e],c2);patch([0 0 1 1-e 0+e 0+e],[0 1 1 1-e 1-e 0+e],c3);plot([0 1 1 0 0],[0 0 1 1 0]);disp('Mux')
  "pd{2,1}" : Outport
      mask Display: e = 0.06;c1 = [120 230 180]/255;c2 = ([120 230 180]+0)/(256+128);c3 = ([120 230 180]+128)/(256+128);patch([0 1 1 0],[0 0 1 1],c1);patch([0 1 1 1-e 1-e 0+e],[0 0 1 1-e 0+e 0+e],c2);patch([0 0 1 1-e 0+e 0+e],[0 1 1 1-e 1-e 0+e],c3);plot([0 1 1 0 0],[0 0 1 1 0]);
  wires:
  "p{2}"/1 -> mux/1
  mux/1 -> "pd{2,1}"/1
